simulink model "LACS"  (R2016b)
settings: Solver=VariableStepAuto  StartTime=0.0  StopTime=10  RelTol=1e-3
values from neighbouring files (symbols this model uses):
  coefficient = 0.8    [LACS.sldd]
  Detal_ref = 0.00022116955850615819 0.00022116955850615819 0.00024339323736781077 0.00026784369743330114 0.00029474273075037104 0.00032433393975435165 0.00035688482250496254 0.00039268904453642435 0.00043206891122917146 0.00047537805500027884 0.00052300435183202216 0.00057537308165349073 0.00063295034678974044 0.00069624676200566427 0.00076582142849131239 0.0008422862023284908 0.000926310265386283 0.0010186250    [LACS.sldd]    (also in path_generate.m = zeros(N,1))
  driver_decel = 4.0    [LACS.sldd]
  EgoLength = 3.048    [LACS.sldd]
  egopath = 0.0 0.25 0.5 0.75 1.0 1.25 1.5 1.7500000000000002 2.0 2.25 2.5 2.75 3.0 3.25 3.5000000000000004 3.75 4.0 4.25 4.5 4.75 5.0 5.25 5.5 5.75 6.0 6.25 6.5 6.75 7.0000000000000009 7.2499999999999991 7.5 7.75 8.0 8.25 8.5 8.75 9.0 9.25 9.5 9.75 10.0 10.25 10.5 10.75 11.0 11.25 11.5 11.75 12.0 12.25 12.5 12.75 13.0 13.25 13.5 13.750000000000002 14.000000000000002 14.250000000000002 14.499999999999998 14.7    [LACS.sldd]
  egoSpdLimit_H = 150.0    [LACS.sldd]
  egoSpdLimit_L = 10.0    [LACS.sldd]
  EgoWidth = 1.628    [LACS.sldd]
  ESA_Active = 3.0    [LACS.sldd]
  ESA_mask_1 = 31.0    [LACS.sldd]
  ESA_mask_2 = 15.0    [LACS.sldd]
  ESA_mask_3 = 255.0    [LACS.sldd]
  ESA_mask_4 = 31.0    [LACS.sldd]
  ESA_Passive = 1.0    [LACS.sldd]
  ESA_Standby = 2.0    [LACS.sldd]
  g = 9.8    [LACS.sldd]
  headwayoffset = 1.524    [LACS.sldd]
  LatAccelThershold = 0.05    [LACS.sldd]
  LatDis = 0.5    [LACS.sldd]
  LatSafetyThershold = 0.5    [LACS.sldd]
  LengthObj = 3.0    [LACS.sldd]
  ObjWidth = 2.0    [LACS.sldd]
  PB1_decel = 3.0    [LACS.sldd]
  PB2_decel = 5.0    [LACS.sldd]
  PB3_decel = 8.0    [LACS.sldd]
  Phi_dot_ref = 0.00085065224568106894 0.00085065224568106894 0.000936127966106986 0.0010301682404378703 0.0011336261186052523 0.0012474385378394444 0.001372634343205976 0.0015103430260158721 0.001661804233646022 0.0018283781058153412 0.0020115564932359636 0.0022129751145658549 0.0024344267064660809 0.0026778752189651235 0.0029454711038487576 0.0032395677369184911 0.0035627390050890382 0.0039177980756855638 0.004    [LACS.sldd]    (also in path_generate.m = zeros(N,1))
  Phi_ref = 0.00038406250525431664 0.00042271073336932769 0.00046524334565338114 0.00051204974395873044 0.000563558155980624 0.00062023946191088657 0.00068261138880285879 0.00075124310596315759 0.0008267602572639512 0.0009098504689462523 0.0010012693742370194 0.0011018471988988175 0.0012124959546271103 0.0013342172899504143 0.0014681110508986705 0.0016153846060911084 0.0017773629929370329 0.001955499943191484    [LACS.sldd]    (also in path_generate.m = phi_ref)
  SteerAngleLimit = 20.0    [LACS.sldd]
  SteerAngleSpdLimit = 20.0    [LACS.sldd]
  StrAngSpdThershold = 0.05    [LACS.sldd]
  StrAngThershold = 0.0    [LACS.sldd]
  Time2React = 1.2    [LACS.sldd]
  timeMargin = 0.5    [LACS.sldd]
  TTCthreshold1 = 2.5    [LACS.sldd]
  TTCthreshold3 = 1.0    [LACS.sldd]
  X_dot_ref = 10.0 10.0 10.0 9.9999999999999947 10.0 10.0 10.0 10.0 10.0 10.0 10.0 10.0 10.0 10.0 10.0 10.000000000000018 10.0 10.0 10.0 10.0 10.0 10.0 10.0 10.0 10.0 10.0 10.0 10.0 10.0 10.0 10.0 10.0 10.0 10.0 10.0 10.0 10.0 10.0 10.0 10.0 10.0 10.0 10.0 10.0 10.0 10.0 10.0 10.0 10.0 10.0 10.0 10.0 10.0 10.0 10.0 10.0 10.0 10.0 10.0 10.0 10.0 10.0 10.0 9.9999999999999289 10.0 10.0 10.0 10.0 10.0 10.0 10.0 10.    [LACS.sldd]    (also in path_generate.m = zeros(N,1))
  X_ref = 0.05 0.55 1.05 1.55 2.05 2.55 3.05 3.55 4.05 4.55 5.05 5.55 6.05 6.55 7.05 7.55 8.05 8.55 9.05 9.55 10.05 10.55 11.05 11.55 12.05 12.55 13.05 13.55 14.05 14.55 15.05 15.55 16.05 16.55 17.05 17.55 18.05 18.55 19.05 19.55 20.05 20.55 21.05 21.55 22.05 22.55 23.05 23.55 24.05 24.55 25.05 25.55 26.05 26.55 27.05 27.55 28.05 28.55 29.05 29.55 30.05 30.55 31.05 31.55 32.05 32.55 33.05 33.55 34.05 34.55    [LACS.sldd]    (also in path_generate.m = X_phi')
  Y_dot_ref = 0.0044363771042237217 0.0044363771042237217 0.00488273213335339 0.0053739322979981 0.0059144698111347933 0.0065092840662692251 0.0071638055584438178 0.0078840039934084845 0.0086764409570179273 0.0095483275445279979 0.01050758737719603 0.011562925461771293 0.012723903376023141 0.014001021290828194 0.015405807364013962 0.016950915064438028 0.018650229002128878 0.020518979854070446 0.0225738689793052    [LACS.sldd]    (also in path_generate.m = zeros(N,1))
  Y_ref = 0.0020016327462461514 0.0022031718511841521 0.0024249907063953382 0.0026691273130630077 0.0029378239279629127 0.0032335474185196523 0.0035590116218331136 0.0039172018997553045 0.0043114020994257287 0.0047452241472766251 0.005222640524503025 0.0057480198933628265 0.0063261661664513911 0.0069623613352525482 0.0076624123997939579 0.008432702767994656 0.0092802485212165574 0.010212759971323001 0.01123    [LACS.sldd]    (also in path_generate.m = zeros(N,1))
undefined symbols (not defined in the file or in its folder): ADR_ADRCycleTime, ADR_SteeringYawrateThresh_p, AEB_mask1, aubr, CAEB_AccelPdlPosLimit, CAEB_AccelPdlPosSpdThreshold, CAEB_CalAEBLongVelObjLimit_mps, CAEB_CalAEBVMaxDec_kmph, ESA_AESACTIVE, ESA_ERROR, ESA_ESAFunctionOFF, ESA_ESAFunctionON, ESA_ESASwichOFF, ESA_ESS_DriverSteeringNumThreshold, ESA_ESSACTIVE, ESA_ForewardCollissionLevel2, ESA_ForewardCollissionLevel3, ESA_OFF, ESA_PASSIVE, ESA_PLAN_AES, ESA_PLAN_ESSLEFT, ESA_PLAN_ESSRIGHT, ESA_PLAN_FAILURE, ESA_PLAN_OFF, ESA_PLAN_STANDBY, ESA_PLAN_WAIT, ESA_SPEEDLIMITH6_p, ESA_SPEEDLIMITH7_p, ESA_SPEEDLIMITL6_p, ESA_SPEEDLIMITL7_p, ESA_STANDBY, ESA_StrAngSpdT6_p, FromAngle2Rad, Kp, magnitude, tablebr, TTCthreshold, vubr
libraries: simulink x15, Solver_SF x9, simulink_extras x1
(part 5 of 5)

== matlab function LACS/Planning&Controlling/findLookaheadPoint ==
  data: pos input; v input; RefPos input; lookaheadPoint output; idx_target output; Kv input; Ld0 input
function [lookaheadPoint,idx_target] = findLookaheadPoint(pos,v,RefPos,Kv,Ld0)

% 找到距离当前位置最近的一个参考轨迹点的序号,把每一个点与起始点的距离都计算一遍并存到dist矩阵里面，在找到最小的距离即可
sizeOfRefPos = size(RefPos,1);
for i = 1:sizeOfRefPos
    dist(i,1) = norm(RefPos(i,:) - pos);
end
[~,idx] = min(dist);

% 从该点开始向轨迹前方搜索，找到与预瞄距离最相近的一个轨迹点
L_step = 0;     %参考轨迹上几个相邻点的累计距离
Ld = Kv * v + Ld0;      %Ld0是预瞄距离的下限值
while L_step < Ld && idx < sizeOfRefPos
    L_step = L_step + norm(RefPos(idx + 1,:) - RefPos(idx,:));
    idx = idx + 1;
end
idx_target = idx;
lookaheadPoint = RefPos(idx,:);
end

== matlab function LACS/trajectoryPlanning3 ==
  data: ld_pre output; ld_veh input; refpath input; currentPose input; currentPose output
function [ld_pre,currentPose]  = fcn(ld_veh,refpath,currentPose)
ld_pre = zeros(length(refpath),1);
currentPose_X = currentPose(1);
currentPose_Y = currentPose(2);
 for i = 1 : length(refpath)
  currentPose_X = refpath(i);
  ld_pre(i) = ld_veh + currentPose_Y;
  currentPose_Y = ld_pre(i) + currentPose_Y;
 end
  currentPose(1) = currentPose_X;
  currentPose(2) = currentPose_Y;
end

== stateflow chart LACS/ESAsts/ESA stateflow ==
  state ESA_ON
    state Passive
      en,du:
      ESAsts = ESA_Passive;
    state Standby
      en,du:
      ESAsts = ESA_Standby;
    state Active
      en,du:
      ESAsts = ESA_Active;
    (default) -> Passive
    Passive -> Standby : [fc1==1]
    Standby -> Passive [order 2] : [fc1~=1&fc2==1]
    Standby -> Active [order 1] : [fc3==1]
    Active -> Passive : [fc4==1]
  (default) -> ESA_ON
  data: ESAsts output; fc1 input boolean; fc2 input boolean; fc3 input boolean; fc4 input boolean; ESA_Passive parameter; ESA_Standby parameter; ESA_Active parameter

== matlab function LACS/trajectoryPlanning5 ==
  data: v_x input; ye input; te input; egopath_x output; egopath_y output
function [egopath_x,egopath_y] = fcn(v_x,ye,te)

if te<=6
t=0:0.01:te;
egopath = zeros(length(t),2);

for i=1:length(t)
egopath(i,1) = v_x * t(i);
egopath(i,2) = (ye/(te^5)) * (6 * (t(i)^5) - 15 * te * (t(i)^4) + 10 * (te^2) * (t(i)^3));
end
egopath_x = egopath(i,1);
egopath_y = egopath(i,2);
else
egopath_x = 0;
egopath_y = 0;
    
end

== matlab function LACS/trajectoryPlanning1 ==
  data: ld_pre output; ld_veh input; refpath input; currentPose input
function ld_pre  = fcn(ld_veh,refpath,currentPose)
ld_pre = zeros(length(refpath),1);
currentPose = zeros(length(refpath),2);
currentPose_X = currentPose(:,1);
currentPose_Y = currentPose(:,2);
 for i = 1 : length(refpath)
  currentPose_X = refpath(i);
  ld_pre(i) = ld_veh + currentPose_Y(i);
 end
end

== matlab function LACS/trajectoryPlanning2 ==
  data: v_x input; ye input; te input; egopath_x output; egopath_y output
function [egopath_x,egopath_y] = fcn(v_x,ye,te)

t=0:0.01:te;
egopath = zeros(length(t),2);

for i=1:length(t)
egopath(i,1) = v_x * t(i);
egopath(i,2) = (ye/(te^5)) * (6 * (t(i)^5) - 15 * te * (t(i)^4) + 10 * (te^2) * (t(i)^3));
end
egopath_x = egopath(i,1);
egopath_y = egopath(i,2);
   
end

== matlab function LACS/Planning&Controlling/pure_persuit_control ==
  data: lookaheadPoint input; idx_target input; pos input; heading input; v input; RefPos input; delta output; Kv input; Ld0 input; L input
function delta = pure_persuit_control(lookaheadPoint,idx_target,pos,heading,v,RefPos,Kv,Ld0,L)
sizeOfRefPos = size(RefPos,1);
if idx_target < sizeOfRefPos   %如果idx标志小于RefPose的值，则把找到的预瞄点给到临时点，如果大于，则说明已经到底了，则把末端最后一个序列号给到临时点
    Point_temp = lookaheadPoint;
else
    Point_temp = RefPos(end,1:2);
end
alpha = atan2(Point_temp(1,2) - pos(2), Point_temp(1,1) - pos(1)) - heading;    %预瞄距离的直线与x的夹角-航向角
Ld = Kv * v + Ld0;

%前轮转角
delta = atan2(2 * L * sin(alpha), Ld);
end

== matlab function LACS/Planning&Controlling/updatestate ==
  data: a input; pos_old input; heading_old input; v_old input; delta input; wheelbase input; pos_new output; dt input; heading_new output; v_new output
%% 更新状态量
function [pos_new,heading_new,v_new] = updateState(a,pos_old,heading_old,v_old,delta,wheelbase,dt)
pos_new(1) = pos_old(1) + v_old * cos(heading_old) * dt;
pos_new(2) = pos_old(2) + v_old * sin(heading_old) * dt;
heading_new = heading_old + v_old * dt * tan(delta)/wheelbase;
v_new = v_old + a * dt;
end

== matlab function LACS/Planning&Controlling/AccelCaculation ==
  data: Kp input; targetSpeed input; v input; a output; dt input
%% 更新状态量
function a = AccelCaculation(Kp,targetSpeed,v,dt)
a = Kp * (targetSpeed - v)/dt;
end

== matlab function LACS/Planning&Controlling/MATLAB Function ==
  data: RefPos input; pos_actual output; heading_actual output; v_actual output
function [pos_actual,heading_actual,v_actual] = fcn(RefPos)


% 车辆状态初始定义
pos = RefPos(1,:);  %设定起始点，把参考路径第一个点设为当前自车位置
v = 0;
heading = 0;

pos_actual = pos;
heading_actual = heading;
v_actual = v;
idx_target = 1;     %位移的标志位,预瞄点在RefPose里的行号

while idx_target < size(RefPos,1)-1     %当这个标志位达到加载的路径的行数，则退出
    %寻找预瞄距离范围内参考轨迹上距离自车位置最近的路径点
   [lookaheadPoint,idx_target] = findLookaheadPoint(pos,v,RefPos,Kv,Ld0);
   
   %计算控制量
   delta = pure_persuit_control(lookaheadPoint,idx_target,pos,heading,v,RefPos,Kv,Ld0,L);
   
   %计算加速度
   a = Kp * (targetSpeed - v)/dt;   %目标速度-当前速度
   
   %更新状态量
   [pos,heading,v] = updateState(a,pos,heading,v,delta,L,dt);
   
   %保存每一步的实际状态量
   pos_actual(end+1,:) = pos;
   heading_actual(end+1,:) = heading;
   v_actual(end+1,:) = v;  
end

== matlab function LACS/MATLAB Function1 ==
  data: X_ref input; x_ref output; y_ref output; phi_ref output; x_dot_ref output; y_dot_ref output; phi_dot_ref output; detal_ref output; Y_ref input; Phi_ref input; X_dot_ref input; Y_dot_ref input; Phi_dot_ref input; Detal_ref input; x input; y input
function [x_ref,y_ref,phi_ref,x_dot_ref,y_dot_ref,phi_dot_ref,detal_ref]...
    = get_ref_data(X_ref,Y_ref,Phi_ref,X_dot_ref,Y_dot_ref,Phi_dot_ref,Detal_ref,x,y)
    N=size(X_ref,1);
    min_dis=99999;
    index=1;
    for i=1:N
        cur_dis=sqrt( (x-X_ref(i))^2+(y-Y_ref(i))^2 );
        if cur_dis<min_dis
            index=i;
            min_dis=cur_dis;
        end
    end
    [x_ref,y_ref,phi_ref]=deal(X_ref(index),Y_ref(index),Phi_ref(index));
    [x_dot_ref,y_dot_ref,phi_dot_ref]=deal(X_dot_ref(index),Y_dot_ref(index),Phi_dot_ref(index));
    detal_ref=Detal_ref(index);

== matlab function LACS/trajectoryPlanning4 ==
  data: v_x input; ye input; te input; egopath_x output; egopath_y output
function [egopath_x,egopath_y] = fcn(v_x,ye,te)

if te<=20
t=0:0.01:te;
egopath = zeros(length(t),2);

for j=1:length(te)
for i=1:length(t)
egopath(i,1) = v_x * t(i);
egopath(i,2) = (ye/(te(j)^5)) * (6 * (t(i)^5) - 15 * te(j) * (t(i)^4) + 10 * (te(j)^2) * (t(i)^3));
end
egopath_x = egopath(i,1);
egopath_y = egopath(i,2);
end
else
egopath_x = 0;
egopath_y = 0;
end

== matlab function LACS/MATLAB Function2 ==
  data: u input; yaw output
function yaw = angle_norm(u)
while u<-2*pi
    u=u+2*pi;
end
while u>2*pi
    u=u-2*pi;
end
yaw = u;

== matlab function LACS/Planning&Controlling/planning ==
  data: vp output; ap output; t input; xr output; yr output; thetar output; kr output
function [vp,ap,xr,yr,thetar,kr] = fcn(t)
    dx=100; %向前移动100m，向左移动20m，运动时间30s
    dy=10;
    T=30;
    xstart=[0,0,0]; %起点和终点的位置，速度，加速度
    xend=[dx,0,0];
    ystart=[0,0,0];
    yend=[dy,0,0];
    a=zeros(1,6);   %五次多项式有六个系数
    b=zeros(1,6);
    
    %纵向的五次多项式系数
    a(1)=xstart(1);
    a(2)=xstart(2);
    a(3)=xstart(3)/2;
    %求解a(4),a(5),a(6)
    A1=[T^3,T^4,T^5;
        3*T^2,4*T^3,5*T^4;
        6*T,12*T^2,20*T^3];
    B1=[xend(1)-a(1)-a(2)*T-a(3)*T^2;
        xend(2)-a(2)-2*a(3)*T;
        xend(3)-2*a(3)];
    xs=inv(A1)*B1;
    a(4)=xs(1);
    a(5)=xs(2);
    a(6)=xs(3);
    %横向的五次多项式系数
    b(1)=ystart(1);
    b(2)=ystart(2);
    b(3)=ystart(3)/2;
    A2=[dx^3,dx^4,dx^5;
        3*dx^2,4*dx^3,5*dx^4;
        6*dx,12*dx^2,20*dx^3];
    B2=[yend(1)-b(1)-b(2)*dx-b(3)*dx^2;
        yend(2)-b(2)-2*b(3)*dx;
        yend(3)-2*b(3)];
    ys=inv(A2)*B2;
    b(4)=ys(1);
    b(5)=ys(2);
    b(6)=ys(3);
    
    %求解规划轨迹的位置，速度，加速度，曲率
    xr=a(1)+a(2)*t+a(3)*t^2+a(4)*t^3+a(5)*t^4+a(6)*t^5;
    yr=b(1)+b(2)*xr+b(3)*xr^2+b(4)*xr^3+b(5)*xr^4+b(6)*xr^5;
    
    xr_dot=a(2)+2*a(3)*t+3*a(4)*t^2+4*a(5)*t^3+5*a(6)*t^4;
    yr_dx=b(2)+2*b(3)*xr+3*b(4)*xr^2+4*b(5)*xr^3+5*b(6)*xr^4;
    yr_dot=yr_dx*xr_dot;
    
    thetar=atan(yr_dx);
    
    xr_dot2=2*a(3)+6*a(4)*t+12*a(5)*t^2+20*a(6)*t^3;
    yr_dx2=2*b(3)+6*b(4)*xr+12*b(5)*xr^2+20*b(6)*xr^3;
    yr_dot2=yr_dx2*xr_dot^2+yr_dx*xr_dot2;
    
    kr=yr_dx2/((1+yr_dx^2)^1.5);    %曲率
    
    vp=sqrt(xr_dot^2+yr_dot^2);
    
    if xr_dot2>=0
        ap=sqrt(xr_dot2^2+yr_dot2^2);
    else
        ap=-sqrt(xr_dot2^2+yr_dot2^2);
    end

== matlab function LACS/trajectoryPlanning6 ==
  data: v_x input; LatDis input; ObjWidth input; egopath_x output; EgoWidth input; coefficient input; g input; egopath_y output
function [egopath_x,egopath_y] = RefPose(v_x,LatDis,ObjWidth,EgoWidth,coefficient,g)

ye = LatDis + ObjWidth/2 + EgoWidth/2;
te = sqrt((10 * sqrt(3) * ye)/(3 * 0.67 * coefficient * g));

t=0:0.01:te;
RefpathA = zeros(length(t),2);

% for i=1:length(t)
% Refpath(i,1) = v_x * t(i);
% Refpath(i,2) = (ye/(te^5)) * (6 * (t(i)^5) - 15 * te * (t(i)^4) + 10 * (te^2) * (t(i)^3));
% end

RefpathA(:,1) = v_x * t;
RefpathA(:,2) = (ye/(te^5)) * (6 * (t^5) - 15 * te * (t^4) + 10 * (te^2) * (t^3));

egopath_x = RefpathA(:,1);
egopath_y = RefpathA(:,2);

end

== matlab function LACS/Planning&Controlling/planning1 ==
  data: vp output; ap output; t input; xr output; yr output; thetar output; kr output
function [vp,ap,xr,yr,thetar,kr] = fcn(t)
    LatDis = 0.5;
    ObjWidth = 2.2;
    EgoWidth = 2;
    coefficient = 0.67;
    g = 9.8;
    vx = 25;
    
%     dy = LatDis + ObjWidth/2 + EgoWidth/2;
%     te = sqrt((10 * sqrt(3) * ye)/(3 * 0.67 * coefficient * g));
%     dx=vx * te; %向前移动100m，向左移动20m，运动时间30s
    dy = 2;
    dx = 20;

    xstart=[0,0,0]; %起点和终点的位置，速度，加速度
    xend=[dx,0,0];
    ystart=[0,0,0];
    yend=[dy,0,0];
    a=zeros(1,6);   %五次多项式有六个系数
    b=zeros(1,6);
    
    %纵向的五次多项式系数
    a(1)=xstart(1);
    a(2)=xstart(2);
    a(3)=xstart(3)/2;
    %求解a(4),a(5),a(6)
    A1=[te^3,te^4,te^5;
        3*te^2,4*te^3,5*te^4;
        6*te,12*te^2,20*te^3];
    B1=[xend(1)-a(1)-a(2)*te-a(3)*te^2;
        xend(2)-a(2)-2*a(3)*te;
        xend(3)-2*a(3)];
    xs=inv(A1)*B1;
    a(4)=xs(1);
    a(5)=xs(2);
    a(6)=xs(3);
    %横向的五次多项式系数
    b(1)=ystart(1);
    b(2)=ystart(2);
    b(3)=ystart(3)/2;
    A2=[dx^3,dx^4,dx^5;
        3*dx^2,4*dx^3,5*dx^4;
        6*dx,12*dx^2,20*dx^3];
    B2=[yend(1)-b(1)-b(2)*dx-b(3)*dx^2;
        yend(2)-b(2)-2*b(3)*dx;
        yend(3)-2*b(3)];
    ys=inv(A2)*B2;
    b(4)=ys(1);
    b(5)=ys(2);
    b(6)=ys(3);
    
    %求解规划轨迹的位置，速度，加速度，曲率
    xr=a(1)+a(2)*t+a(3)*t^2+a(4)*t^3+a(5)*t^4+a(6)*t^5;
    yr=b(1)+b(2)*xr+b(3)*xr^2+b(4)*xr^3+b(5)*xr^4+b(6)*xr^5;
    
    xr_dot=a(2)+2*a(3)*t+3*a(4)*t^2+4*a(5)*t^3+5*a(6)*t^4;
    yr_dx=b(2)+2*b(3)*xr+3*b(4)*xr^2+4*b(5)*xr^3+5*b(6)*xr^4;
    yr_dot=yr_dx*xr_dot;
    
    thetar=atan(yr_dx);
    
    xr_dot2=2*a(3)+6*a(4)*t+12*a(5)*t^2+20*a(6)*t^3;
    yr_dx2=2*b(3)+6*b(4)*xr+12*b(5)*xr^2+20*b(6)*xr^3;
    yr_dot2=yr_dx2*xr_dot^2+yr_dx*xr_dot2;
    
    kr=yr_dx2/((1+yr_dx^2)^1.5);    %曲率
    
    vp=sqrt(xr_dot^2+yr_dot^2);
    
    if xr_dot2>=0
        ap=sqrt(xr_dot2^2+yr_dot2^2);
    else
        ap=-sqrt(xr_dot2^2+yr_dot2^2);
    end
